simulink model "ABS_simu"  (R2017b)
settings: Solver=VariableStepAuto  StartTime=0.0  StopTime=30  RelTol=1e-3
values from neighbouring files (symbols this model uses):
  g = 0.5    [ProjetABS.m]
  N = m*grav/4    (= 2452.5)    [ProjetABS.m]
libraries: simulink x2
settings Model: Creator=Table2  LastModifiedBy=Table2

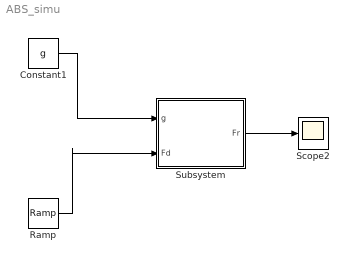
== system ABS_simu ==
  Constant1 : Constant  Value=g
  Ramp : simulink/Sources/Ramp  slope=100  start=0  X0=0
  Scope2 : Scope
  Subsystem : Subsystem
  wires:
  Constant1/1 -> Subsystem/1(g)
  Ramp/1 -> Subsystem/2(Fd)
  Subsystem/1(Fr) -> Scope2/1

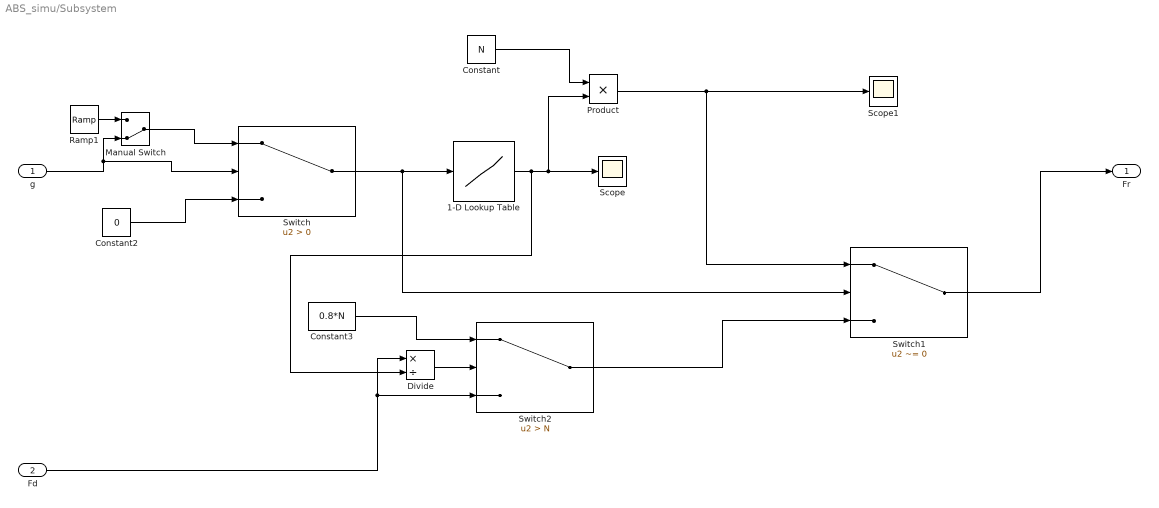
== system ABS_simu/Subsystem ==
  g : Inport
  Fd : Inport  Port=2
  1-D Lookup Table : Lookup_n-D  NumberOfTableDimensions=1  BreakpointsForDimension1=[0,0.18,0.2,0.22,0.25,0.5,0.8,0.9,1]  Table=[0.8,0.94,0.95,0.94,0.85,0.7,0.62,0.61,0.6]  InternalRulePriority=Speed  RndMeth=Simplest  InputSameDT=on
  Constant : Constant  Value=N
  Constant2 : Constant  Value=0
  Constant3 : Constant  Value=0.8*N
  Divide : Product  Inputs=*/
  Manual Switch : ManualSwitch  CurrentSetting=0
  Product : Product
  Ramp1 : simulink/Sources/Ramp  slope=1  start=0  X0=0
  Scope : Scope
  Scope1 : Scope
  Switch : Switch  Criteria=u2 > Threshold
  Switch1 : Switch  Criteria=u2 ~= 0
  Switch2 : Switch  Criteria=u2 > Threshold  Threshold=N
  Fr : Outport
  wires:
  Constant2/1 -> Switch/3
  Fd/1 -> Divide/1, Switch2/3
  Switch1/1 -> Fr/1
  Divide/1 -> Switch2/2
  Product/1 -> Switch1/1, Scope1/1
  Constant/1 -> Product/1
  Switch2/1 -> Switch1/3
  Manual Switch/1 -> Switch/1
  Ramp1/1 -> Manual Switch/1
  Constant3/1 -> Switch2/1
  1-D Lookup Table/1 -> Divide/2, Product/2, Scope/1
  Switch/1 -> Switch1/2, 1-D Lookup Table/1
  g/1 -> Switch/2, Manual Switch/2
